simulink model "P3_Ex11"  (R2021a)
settings: Solver=FixedStepAuto  StartTime=0.0  StopTime=Total_time  RelTol=1e-3  EnableMultiTasking=on
PreLoadFcn:
  | Preload11_12
undefined symbols (not defined in the file): DiscIntNeverNeededParam, K0, Kd, Ki, Kp, Kpot, tau0, Ts
libraries: simulink x3
settings Model: ExtModeTrigDuration=2  Creator=Eneko Lerma  LastModifiedBy=Control Automatic
settings SolverCC: AlgebraicLoopSolver=TrustRegion  AutoInsertRateTranBlk=on
settings DataIOCC: ReturnWorkspaceOutputs=off
settings OptimizationCC: EnhancedBackFolding=on  PassReuseOutputArgsAs=Individual arguments  MaxStackSize=64  OptimizeBlockOrder=speed  DifferentSizesBufferReuse=on  OptimizationCustomize=off  EfficientTunableParamExpr=on
settings DebuggingCC: ParameterPrecisionLossMsg=none  ParameterTunabilityLossMsg=error  SFMachineParentedDataDiag=warning  ArithmeticOperatorsInVariantConditions=warning
settings HardwareCC: ProdBitPerPointer=32  ProdBitPerSizeT=32  ProdBitPerPtrDiffT=32  ProdLargestAtomicInteger=Long  ProdLargestAtomicFloat=Double  ProdWordSize=32  ProdHWDeviceType=ARM Compatible->ARM Cortex
settings SFSimCC: SimUseLocalCustomCode=off  MATLABDynamicMemAlloc=off  CustomCodeUndefinedFunction=UseInterfaceOnly
settings RTWCC: SystemTargetFile=ert.tlc  HardwareBoard=Arduino Due  TemplateMakefile=ert_default_tmf  GenerateReport=on  RTWUseLocalCustomCode=off  Toolchain=Arduino ARM  BuildConfiguration=Faster Runs  IncludeHyperlinkInReport=on  LaunchReport=on  GenerateTraceInfo=on  GenerateTraceReport=on  GenerateTraceReportSl=on  GenerateTraceReportSf=on  GenerateTraceReportEml=on
settings CodeAppCC: ForceParamTrailComments=on  IgnoreCustomStorageClasses=off  OperatorAnnotations=on  SimulinkDataObjDesc=on  SFDataObjDesc=on  InsertBlockDesc=on
settings ERTTargetCC: SupportContinuousTime=on  SupportVariableSizeSignals=on

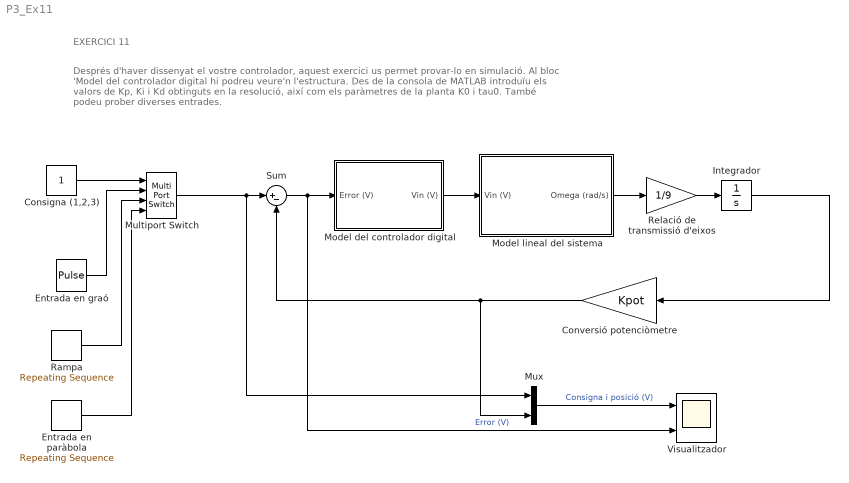
== system P3_Ex11 ==
  note: Després d'haver dissenyat el vostre controlador, aquest exercici us permet provar-lo en simulació. Al bloc 'Model del
      | controlador digital hi podreu veure'n l'estructura. Des de la consola de MATLAB introduïu els valors de Kp, Ki i Kd
      | obtinguts en la resolució, així com els paràmetres de la planta K0 i tau0. També podeu prober diverses entrades.
  note: EXERCICI 11
  Consigna (1,2,3) : Constant
  Conversió potenciòmetre : Gain  Gain=Kpot  OutDataTypeStr=single
  Entrada en paràbola : simulink/Sources/Repeating Sequence  rep_seq_t="[0    0.1000    0.2000    0.3000    0.4000    0.5000    0.6000    0.7000    0.8000 0.9000    1.0000    1.1000    1.2000    1.3000    1.4000    1.5000    1.6000    1.7000 1.8000    1.9000    2.0000    2.1000    2.2000    2.3000    2.4000    2.5000    2.6000 2.7000    2.8000    2.9000    3.0000    3.1000    3.2000    3.3000    3.4000    3.5000\t3.6000    3.7000    3.8000    3.9000    4.0000    4.1000    4.2000    4.3000    4.4000    4.5000    4.6000    4.7000    4.8000    4.9000    5.0000]"  rep_seq_y="[0    0.0008    0.0032    0.0072    0.0128    0.0200    0.0288    0.0392 0.0512    0.0648    0.0800    0.0968    0.1152    0.1352    0.1568    0.1800 0.2048    0.2312    0.2592    0.2888    0.3200    0.3528    0.3872    0.4232 0.4608    0.5000    0.5408    0.5832    0.6272    0.6728    0.7200    0.7688 0.8192    0.8712    0.9248    0.9800    1.0368    1.0952    1.1552    1.2168 1.2800    1.3448    1.4112    1.4792    1.5488    1.6200    1.6928    1.7672 1.8432    1.9208    2.0000]"
  Entrada en graó : DiscretePulseGenerator  PulseType=Time based  Amplitude=2  Period=15  PulseWidth=50
  Integrador : Integrator
  Model del controlador digital : Subsystem
  Model lineal del sistema : Subsystem
  Multiport Switch : MultiPortSwitch  OutDataTypeStr=single
  Mux : Mux  Inputs=2
  Rampa : simulink/Sources/Repeating Sequence  rep_seq_t="[0    0.1000    0.2000    0.3000    0.4000    0.5000    0.6000    0.7000    0.8000 0.9000    1.0000    1.1000    1.2000    1.3000    1.4000    1.5000    1.6000    1.7000 1.8000    1.9000    2.0000    2.1000    2.2000    2.3000    2.4000    2.5000    2.6000 2.7000    2.8000    2.9000    3.0000    3.1000    3.2000    3.3000    3.4000    3.5000\t3.6000    3.7000    3.8000    3.9000    4.0000    4.1000    4.2000    4.3000    4.4000    4.5000    4.6000    4.7000    4.8000    4.9000    5.0000]"  rep_seq_y=[-2.0000,-1.9200,-1.8400,-1.7600,-1.6800,-1.6000,-1.5200,-1.4400,-1.3600,-1.2800,-1.2000,-1.1200,-1.0400,-0.9600,-0.8800,-0.8000,-0.7200,-0.6400,-0.5600,-0.4800,-0.4000,-0.3200,-0.2400,-0.1600,-0.0800,0,0.0800,0.1600,0.2400,0.3200,0.4000,0.4800,0.5600,0.6400,0.7200,0.8000,0.8800,0.9600,1.0400,1.1200,1.2000,1.2800,1.3600,1.4400,1.5200,1.6000,1.6800,1.7600,1.8400,1.9200,2.0000]
  Relació de transmissió d'eixos : Gain  Gain=1/9
  Sum : Sum  Inputs=|+-  AccumDataTypeStr=single
  Visualitzador : Scope  NumInputPorts=2
  wires:
  Mux/1 -> Visualitzador/1  "Consigna i posició (V)"
  Conversió potenciòmetre/1 -> Mux/2, Sum/2
  Multiport Switch/1 -> Sum/1, Mux/1
  Sum/1 -> Model del controlador digital/1(Error (V)), Visualitzador/2  "Error (V)"
  Model del controlador digital/1(Vin (V)) -> Model lineal del sistema/1(Vin (V))
  Consigna (1,2,3)/1 -> Multiport Switch/1
  Entrada en graó/1 -> Multiport Switch/2
  Entrada en paràbola/1 -> Multiport Switch/4
  Rampa/1 -> Multiport Switch/3
  Integrador/1 -> Conversió potenciòmetre/1
  Relació de transmissió d'eixos/1 -> Integrador/1
  Model lineal del sistema/1(Omega (rad/s)) -> Relació de transmissió d'eixos/1

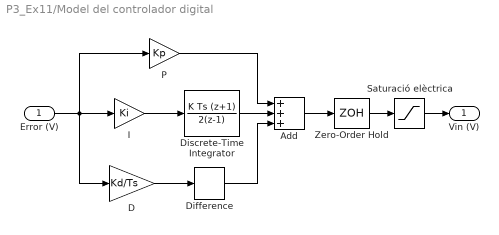
== system P3_Ex11/Model del controlador digital ==
  Error (V) : Inport
  Add : Sum  Inputs=+++  AccumDataTypeStr=single
  D : Gain  Gain=Kd/Ts
  Difference : simulink/Discrete/Difference  ICPrevInput=0.0  OutMin=[]  OutMax=[]  OutDataType=fixdt(1, 16)  OutScaling=2^-10  DoSatur=off
  Discrete-Time Integrator : DiscreteIntegrator  IntegratorMethod=Integration: Trapezoidal  SampleTime=Ts  ICPrevOutput=DiscIntNeverNeededParam  ICPrevScaledInput=DiscIntNeverNeededParam
  I : Gain  Gain=Ki
  P : Gain  Gain=Kp
  Saturació elèctrica : Saturate  UpperLimit=5  LowerLimit=-5
  Zero-Order Hold : ZeroOrderHold  SampleTime=Ts
  Vin (V) : Outport  VectorParamsAs1DForOutWhenUnconnected=off
  wires:
  Difference/1 -> Add/3
  Discrete-Time Integrator/1 -> Add/2
  Add/1 -> Zero-Order Hold/1
  Error (V)/1 -> P/1, I/1, D/1
  I/1 -> Discrete-Time Integrator/1
  P/1 -> Add/1
  D/1 -> Difference/1
  Zero-Order Hold/1 -> Saturació elèctrica/1
  Saturació elèctrica/1 -> Vin (V)/1

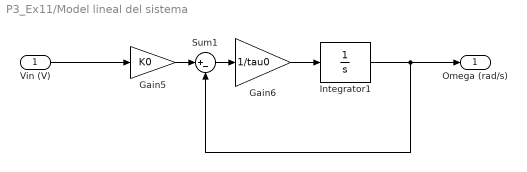
== system P3_Ex11/Model lineal del sistema ==
  Vin (V) : Inport
  Gain5 : Gain  Gain=K0
  Gain6 : Gain  Gain=1/tau0
  Integrator1 : Integrator
  Sum1 : Sum  Inputs=|+-
  Omega (rad/s) : Outport  VectorParamsAs1DForOutWhenUnconnected=off
  wires:
  Gain6/1 -> Integrator1/1
  Gain5/1 -> Sum1/1
  Sum1/1 -> Gain6/1
  Vin (V)/1 -> Gain5/1
  Integrator1/1 -> Omega (rad/s)/1, Sum1/2
